simulink model "CMState"  (R2017b)
settings: Solver=VariableStepAuto  StartTime=0.0  StopTime=5  RelTol=1e-3
undefined symbols (not defined in the file or in its folder): Yo
settings Model: Creator=benma  LastModifiedBy=benma

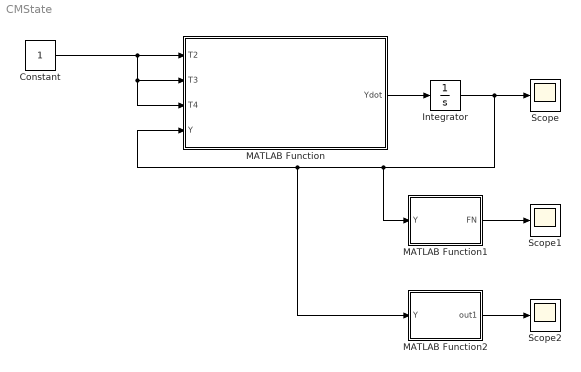
== system CMState ==
  Constant : Constant
  Integrator : Integrator  InitialCondition=Yo
  MATLAB Function : MATLAB Function  TreatAsAtomicUnit=on
  MATLAB Function1 : MATLAB Function  TreatAsAtomicUnit=on
  MATLAB Function2 : MATLAB Function  TreatAsAtomicUnit=on
  Scope : Scope
  Scope1 : Scope
  Scope2 : Scope
  wires:
  Integrator/1 -> Scope/1, MATLAB Function1/1(Y), MATLAB Function2/1(Y), MATLAB Function/4(Y)
  Constant/1 -> MATLAB Function/3(T4), MATLAB Function/2(T3), MATLAB Function/1(T2)
  MATLAB Function/1(Ydot) -> Integrator/1
  MATLAB Function1/1(FN) -> Scope1/1
  MATLAB Function2/1(out1) -> Scope2/1

== matlab function CMState/MATLAB Function ==
  data: T2 input; Ydot output; T3 input; T4 input; Y input
function Ydot = System1_ground(T2,T3,T4,Y)
%SYSTEM1_GROUND
%    OUT1 = SYSTEM1_GROUND(T2,T3,T4,Y)

%    This function was generated by the Symbolic Math Toolbox version 8.0.
%    22-Oct-2018 10:53:19

t2 = Y(2);
t3 = t2.*2.0;
t4 = Y(3);
t5 = t4.*2.0;
t6 = Y(4);
t7 = t6.*2.0;
t8 = Y(1);
t9 = Y(6);
t10 = t9.^2;
t11 = t2-t4;
t12 = sin(t11);
t13 = Y(7);
t14 = Y(8);
t15 = t2+t5;
t16 = sin(t15);
t17 = t13.^2;
t18 = t2-t7;
t19 = sin(t18);
t20 = t2+t7;
t21 = sin(t20);
t22 = cos(t5);
t23 = cos(t7);
t24 = -t2+t4+t7;
t25 = sin(t24);
t26 = t14.^2;
t27 = t2+t5+t7;
t28 = sin(t27);
t29 = cos(t15);
t30 = cos(t11);
t31 = cos(t18);
t32 = cos(t20);
t33 = cos(t27);
t34 = cos(t24);
t35 = t2+t4+t6;
t36 = sin(t35);
t37 = Y(9);
t38 = t3+t5;
t39 = t3-t7;
t40 = t3+t7;
t41 = t3+t5+t7;
t42 = sin(t2);
t43 = t5+t7;
t44 = cos(t43);
t45 = t2+t4;
t46 = sin(t45);
t47 = cos(t2);
t48 = -t2+t4+t6;
t49 = sin(t48);
t50 = t2-t4+t6;
t51 = sin(t50);
t52 = t2+t4-t6;
t53 = sin(t52);
t54 = t2+t4+t7;
t55 = sin(t54);
t56 = t37.^2;
t57 = cos(t45);
t58 = cos(t54);
t59 = cos(t41);
t60 = cos(t3);
t61 = cos(t38);
t62 = t61.*8.1e1;
t63 = cos(t39);
t64 = t63.*8.1e1;
t65 = cos(t40);
t66 = t65.*8.1e1;
t67 = t44.*4.5e1;
t191 = t59.*9.0;
t192 = t60.*6.57e2;
t193 = t22.*4.05e2;
t194 = t23.*3.33e2;
t68 = t62+t64+t66+t67-t191-t192-t193-t194+1.31e3;
t69 = 1.0./t68;
t70 = t5+t7-t8;
t71 = cos(t70);
t72 = cos(t8);
t73 = t3+t8;
t74 = cos(t73);
t75 = t74.*1.074195e5;
t76 = -t5+t8;
t77 = cos(t76);
t78 = t77.*3.97305e4;
t79 = t5+t8;
t80 = cos(t79);
t81 = t80.*3.97305e4;
t82 = -t7+t8;
t83 = cos(t82);
t84 = t83.*3.09015e4;
t85 = t7+t8;
t86 = cos(t85);
t87 = t86.*3.09015e4;
t88 = t3+t5+t8;
t89 = cos(t88);
t90 = t3-t7+t8;
t91 = cos(t90);
t92 = t3+t7+t8;
t93 = cos(t92);
t94 = t5+t7+t8;
t95 = cos(t94);
t96 = t3+t5+t7+t8;
t97 = cos(t96);
t98 = t97.*1.4715e3;
t99 = sin(t3);
t100 = sin(t5);
t101 = t10.*t12.*5.4e3;
t102 = t12.*t17.*5.4e3;
t103 = t12.*t26.*5.4e3;
t104 = t3+t4;
t105 = sin(t104);
t106 = t4-t6;
t107 = sin(t106);
t108 = t4+t7;
t109 = sin(t108);
t110 = T2.*t22.*8.1e3;
t111 = t10.*t25.*4.5e2;
t112 = t17.*t25.*4.5e2;
t113 = t3+t4-t6;
t114 = sin(t113);
t115 = t25.*t26.*4.5e2;
t116 = t3+t4+t7;
t117 = sin(t116);
t118 = t17.*t28.*1.5e2;
t119 = T3.*t30.*1.62e4;
t120 = cos(t104);
t121 = cos(t108);
t122 = T3.*t33.*9.0e2;
t123 = T4.*t34.*2.7e3;
t124 = cos(t116);
t125 = t10.*t36.*5.0e1;
t126 = t17.*t36.*5.0e1;
t127 = t26.*t36.*5.0e1;
t128 = t36.*t56.*5.0e1;
t129 = sin(t38);
t130 = sin(t39);
t131 = sin(t40);
t132 = sin(t43);
t133 = sin(t41);
t134 = t10.*t133.*1.5e2;
t135 = cos(t35);
t136 = t17.*t42.*1.87e4;
t137 = sin(t4);
t138 = t10.*t46.*3.15e3;
t139 = t17.*t46.*3.15e3;
t140 = t26.*t46.*3.15e3;
t141 = t4+t6;
t142 = sin(t141);
t143 = T3.*t47.*1.92e4;
t144 = cos(t4);
t145 = t10.*t51.*1.35e3;
t146 = t10.*t53.*9.0e2;
t147 = t17.*t51.*1.35e3;
t148 = t17.*t53.*9.0e2;
t149 = t26.*t51.*1.35e3;
t150 = t26.*t53.*9.0e2;
t151 = t3+t4+t6;
t152 = sin(t151);
t153 = t51.*t56.*1.35e3;
t154 = t53.*t56.*9.0e2;
t155 = T4.*t57.*1.35e4;
t156 = T3.*t58.*1.8e3;
t157 = cos(t48);
t158 = T4.*t157.*3.6e3;
t159 = cos(t50);
t160 = cos(t52);
t161 = T4.*t160.*5.4e3;
t162 = t9.*t13.*t46.*6.3e3;
t163 = t9.*t14.*t46.*6.3e3;
t164 = t13.*t14.*t46.*6.3e3;
t165 = t9.*t13.*t51.*2.7e3;
t166 = t9.*t13.*t53.*1.8e3;
t167 = t9.*t14.*t51.*2.7e3;
t168 = t9.*t14.*t53.*1.8e3;
t169 = t9.*t37.*t51.*2.7e3;
t170 = t13.*t14.*t51.*2.7e3;
t171 = t9.*t37.*t53.*1.8e3;
t172 = t13.*t14.*t53.*1.8e3;
t173 = t13.*t37.*t51.*2.7e3;
t174 = t13.*t37.*t53.*1.8e3;
t175 = t14.*t37.*t51.*2.7e3;
t176 = t14.*t37.*t53.*1.8e3;
t177 = t9.*t12.*t13.*1.08e4;
t178 = t9.*t12.*t14.*1.08e4;
t179 = t12.*t13.*t14.*1.08e4;
t180 = t9.*t13.*t25.*9.0e2;
t181 = t9.*t14.*t25.*9.0e2;
t182 = t9.*t13.*t28.*3.0e2;
t183 = t13.*t14.*t25.*9.0e2;
t184 = t9.*t13.*t36.*1.0e2;
t185 = t9.*t14.*t36.*1.0e2;
t186 = t9.*t36.*t37.*1.0e2;
t187 = t13.*t14.*t36.*1.0e2;
t188 = t13.*t36.*t37.*1.0e2;
t189 = t14.*t36.*t37.*1.0e2;
t190 = t9.*t13.*t42.*3.74e4;
t195 = t2+t8;
t196 = cos(t195);
t197 = t196.*1.702035e5;
t198 = t2+t5+t8;
t199 = cos(t198);
t200 = t2-t7+t8;
t201 = cos(t200);
t202 = t2+t7+t8;
t203 = cos(t202);
t204 = t2+t5+t7+t8;
t205 = cos(t204);
t206 = t205.*2.943e3;
t207 = -t2+t8;
t208 = cos(t207);
t209 = t2+t5-t8;
t210 = cos(t209);
t211 = t210.*3.97305e4;
t212 = t2+t7-t8;
t213 = cos(t212);
t214 = t213.*2.6487e4;
t215 = -t2+t7+t8;
t216 = cos(t215);
t217 = t216.*2.6487e4;
t218 = t2+t5+t7-t8;
t219 = cos(t218);
t220 = t10.*t99.*1.095e4;
t221 = t17.*t99.*1.095e4;
t222 = sin(t7);
t223 = t26.*t105.*5.4e3;
t224 = t3+t6;
t225 = sin(t224);
t226 = t5+t6;
t227 = sin(t226);
t228 = t26.*t109.*1.2e3;
t229 = t10.*t114.*1.35e3;
t230 = t17.*t114.*1.35e3;
t231 = t26.*t114.*1.35e3;
t232 = t3+t5+t6;
t233 = sin(t232);
t234 = t56.*t114.*1.35e3;
t235 = T2.*t29.*8.1e3;
t236 = T2.*t31.*2.7e3;
t237 = T2.*t32.*2.7e3;
t238 = T4.*t120.*1.62e4;
t239 = cos(t106);
t240 = T4.*t121.*7.2e3;
t241 = cos(t113);
t242 = T4.*t241.*8.1e3;
t243 = t3-t6;
t244 = sin(t243);
t245 = t10.*t132.*7.5e2;
t246 = t17.*t132.*7.5e2;
t247 = sin(t6);
t248 = T2.*t61.*8.1e3;
t249 = t10.*t152.*3.0e2;
t250 = t17.*t152.*3.0e2;
t251 = t26.*t152.*3.0e2;
t252 = t56.*t152.*3.0e2;
t253 = cos(t141);
t254 = T4.*t253.*1.41e4;
t255 = cos(t151);
t256 = t9.*t13.*t152.*6.0e2;
t257 = t9.*t14.*t152.*6.0e2;
t258 = t9.*t37.*t152.*6.0e2;
t259 = t13.*t14.*t152.*6.0e2;
t260 = t13.*t37.*t152.*6.0e2;
t261 = t14.*t37.*t152.*6.0e2;
t262 = t9.*t13.*t99.*2.19e4;
t263 = t9.*t14.*t105.*1.08e4;
t264 = t13.*t14.*t105.*1.08e4;
t265 = t9.*t14.*t109.*2.4e3;
t266 = t13.*t14.*t109.*2.4e3;
t267 = t9.*t13.*t114.*2.7e3;
t268 = t9.*t14.*t114.*2.7e3;
t269 = t9.*t37.*t114.*2.7e3;
t270 = t13.*t14.*t114.*2.7e3;
t271 = t13.*t37.*t114.*2.7e3;
t272 = t14.*t37.*t114.*2.7e3;
t273 = t9.*t13.*t132.*1.5e3;
t274 = t2+t4+t7+t8;
t275 = cos(t274);
t276 = t275.*1.4715e3;
t277 = t2+t4-t8;
t278 = cos(t277);
t279 = t278.*3.97305e4;
t280 = -t2+t4+t8;
t281 = cos(t280);
t282 = t2-t4+t8;
t283 = cos(t282);
t284 = t283.*5.2974e4;
t285 = t2+t4+t7-t8;
t286 = cos(t285);
t287 = -t2+t4+t7+t8;
t288 = cos(t287);
t289 = t288.*1.32435e4;
t290 = t2-t4-t7+t8;
t291 = cos(t290);
t292 = t2+t4+t8;
t293 = cos(t292);
t294 = t10.*t12.*1.35e4;
t295 = t10.*t25.*2.25e3;
t296 = t56.*t233.*4.5e2;
t297 = T2.*t120.*1.62e4;
t298 = T2.*t121.*7.2e3;
t299 = cos(t224);
t300 = cos(t226);
t301 = T2.*t34.*2.7e3;
t302 = cos(t232);
t303 = T3.*t124.*2.7e3;
t304 = t10.*t129.*1.35e3;
t305 = t17.*t129.*1.35e3;
t306 = t26.*t129.*1.35e3;
t307 = t56.*t244.*3.15e3;
t308 = t56.*t247.*1.19e4;
t309 = cos(t243);
t310 = T4.*t44.*4.5e3;
t311 = T3.*t59.*9.0e2;
t312 = T3.*t144.*2.97e4;
t313 = cos(t6);
t314 = t10.*t55.*6.0e2;
t315 = T2.*t57.*1.35e4;
t316 = t9.*t37.*t233.*9.0e2;
t317 = t13.*t37.*t233.*9.0e2;
t318 = t14.*t37.*t233.*9.0e2;
t319 = t9.*t13.*t129.*2.7e3;
t320 = t9.*t14.*t129.*2.7e3;
t321 = t13.*t14.*t129.*2.7e3;
t322 = t9.*t37.*t244.*6.3e3;
t323 = t13.*t37.*t244.*6.3e3;
t324 = t14.*t37.*t244.*6.3e3;
t325 = t9.*t37.*t247.*2.38e4;
t326 = t13.*t37.*t247.*2.38e4;
t327 = t14.*t37.*t247.*2.38e4;
Ydot = [t9;t13;t14;t37;Y(10);t69.*(T2.*-1.69e4-t71.*4.4145e3-t72.*2.418165e5+t75+t78+t81+t84+t87-t89.*1.32435e4-t91.*1.32435e4-t93.*1.32435e4-t95.*4.4145e3+t98+t101+t102+t103+t110+t111+t112+t115+t118+t119+t122+t123+t125+t126+t127+t128+t134+t136+t138+t139+t140+t143+t145+t146+t147+t148+t149+t150+t153+t154+t155+t156+t158+t161+t162+t163+t164+t165+t166+t167+t168+t169+t170+t171+t172+t173+t174+t175+t176+t177+t178+t179+t180+t181+t182+t183+t184+t185+t186+t187+t188+t189+t190+t220+t235+t236+t237+T2.*t23.*4.5e3-T3.*t29.*8.1e3-T3.*t31.*2.7e3-T4.*t30.*1.62e4-T2.*t33.*9.0e2-T3.*t32.*2.7e3-T3.*t34.*2.7e3-T2.*t44.*9.0e2-T2.*t47.*1.92e4-T3.*t57.*1.35e4-T4.*t58.*1.8e3-T4.*t135.*1.5e3-T4.*t159.*8.1e3-t10.*t16.*1.35e3-t10.*t19.*2.25e3-t10.*t21.*2.25e3-t16.*t17.*1.35e3-t17.*t19.*2.25e3+t10.*t28.*1.5e2-t17.*t21.*2.25e3+t10.*t42.*1.87e4-t10.*t49.*3.0e2-t10.*t55.*3.0e2-t17.*t49.*3.0e2-t17.*t55.*3.0e2-t26.*t49.*3.0e2-t26.*t55.*3.0e2-t49.*t56.*3.0e2-t10.*t129.*1.35e3-t10.*t130.*1.35e3-t10.*t131.*1.35e3-t9.*t13.*t16.*2.7e3-t9.*t13.*t19.*4.5e3-t9.*t13.*t21.*4.5e3-t9.*t13.*t49.*6.0e2-t9.*t14.*t49.*6.0e2-t13.*t14.*t49.*6.0e2-t9.*t13.*t55.*6.0e2-t9.*t14.*t55.*6.0e2-t13.*t14.*t55.*6.0e2-t9.*t37.*t49.*6.0e2-t13.*t37.*t49.*6.0e2-t14.*t37.*t49.*6.0e2).*(3.0./5.0e1);t69.*(T2.*-4.76e4+T3.*3.07e4-t71.*4.4145e3-t72.*2.418165e5+t75+t78+t81+t84+t87-t89.*1.32435e4-t91.*1.32435e4-t93.*1.32435e4-t95.*4.4145e3+t98+t101+t102+t103+t110+t111+t112+t115+t118+t119+t122+t123+t125+t126+t127+t128+t134+t136+t138+t139+t140+t143+t145+t146+t147+t148+t149+t150+t153+t154+t155+t156+t158+t161+t162+t163+t164+t165+t166+t167+t168+t169+t170+t171+t172+t173+t174+t175+t176+t177+t178+t179+t180+t181+t182+t183+t184+t185+t186+t187+t188+t189+t190+t197-t199.*2.6487e4-t201.*2.20725e4-t203.*2.20725e4+t206-t208.*2.015955e5+t211+t214+t217-t219.*4.4145e3+t221+t223+t228+t229+t230+t231+t234+t238+t240+t242+t245+t246+t248+t249+t250+t251+t252+t254+t256+t257+t258+t259+t260+t261+t262+t263+t264+t265+t266+t267+t268+t269+t270+t271+t272+t273+t303+t311+t312+T2.*t23.*1.44e4-T3.*t23.*9.9e3+T2.*t29.*1.62e4-T3.*t29.*8.1e3+T2.*t31.*5.4e3+T2.*t32.*5.4e3-T3.*t31.*2.7e3-T4.*t30.*1.62e4-T2.*t33.*1.8e3-T3.*t32.*2.7e3-T3.*t34.*2.7e3-T2.*t44.*9.0e2-T2.*t47.*3.84e4-T3.*t57.*1.35e4-T2.*t59.*9.0e2-T4.*t58.*1.8e3-T3.*t61.*8.1e3-T3.*t120.*1.62e4-T3.*t121.*7.2e3-T4.*t124.*2.7e3-T4.*t135.*1.5e3-T4.*t144.*2.97e4-T4.*t159.*8.1e3-T4.*t239.*2.16e4-T4.*t255.*3.6e3-t10.*t16.*8.1e3-t10.*t19.*7.2e3-t10.*t21.*7.2e3-t16.*t17.*1.35e3-t17.*t19.*2.25e3+t10.*t28.*9.0e2-t17.*t21.*2.25e3+t10.*t42.*5.66e4-t10.*t49.*3.0e2-t10.*t55.*3.0e2-t17.*t49.*3.0e2-t17.*t55.*3.0e2-t26.*t49.*3.0e2-t26.*t55.*3.0e2-t49.*t56.*3.0e2+t10.*t99.*2.19e4-t10.*t100.*6.75e3+t10.*t105.*5.4e3-t10.*t107.*3.6e3-t17.*t100.*6.75e3+t10.*t109.*1.2e3+t17.*t105.*5.4e3-t17.*t107.*3.6e3+t17.*t109.*1.2e3-t10.*t117.*4.5e2-t26.*t107.*3.6e3-t17.*t117.*4.5e2-t10.*t129.*1.35e3-t10.*t130.*2.7e3-t10.*t131.*2.7e3-t26.*t117.*4.5e2-t10.*t137.*1.665e4-t17.*t130.*1.35e3-t17.*t131.*1.35e3-t10.*t142.*1.55e3-t17.*t137.*1.665e4-t17.*t142.*1.55e3-t26.*t137.*1.665e4-t56.*t107.*3.6e3-t26.*t142.*1.55e3-t56.*t142.*1.55e3-t9.*t13.*t16.*2.7e3-t9.*t13.*t19.*4.5e3-t9.*t13.*t21.*4.5e3-t9.*t13.*t49.*6.0e2-t9.*t14.*t49.*6.0e2-t13.*t14.*t49.*6.0e2-t9.*t13.*t55.*6.0e2-t9.*t14.*t55.*6.0e2-t13.*t14.*t55.*6.0e2-t9.*t37.*t49.*6.0e2-t13.*t37.*t49.*6.0e2-t14.*t37.*t49.*6.0e2-t9.*t13.*t100.*1.35e4+t9.*t13.*t105.*1.08e4-t9.*t13.*t107.*7.2e3-t9.*t14.*t107.*7.2e3+t9.*t13.*t109.*2.4e3-t13.*t14.*t107.*7.2e3-t9.*t13.*t117.*9.0e2-t9.*t14.*t117.*9.0e2-t13.*t14.*t117.*9.0e2-t9.*t13.*t130.*2.7e3-t9.*t13.*t131.*2.7e3-t9.*t37.*t107.*7.2e3-t13.*t37.*t107.*7.2e3-t14.*t37.*t107.*7.2e3-t9.*t13.*t137.*3.33e4-t9.*t14.*t137.*3.33e4-t9.*t13.*t142.*3.1e3-t13.*t14.*t137.*3.33e4-t9.*t14.*t142.*3.1e3-t13.*t14.*t142.*3.1e3-t9.*t37.*t142.*3.1e3-t13.*t37.*t142.*3.1e3-t14.*t37.*t142.*3.1e3).*(-3.0./5.0e1);t69.*(T2.*-3.07e4+T3.*8.06e4-T4.*4.99e4+t197-t199.*2.6487e4-t201.*2.20725e4-t203.*2.20725e4+t206-t208.*2.015955e5+t211+t214+t217-t219.*4.4145e3+t220+t221+t223+t228+t229+t230+t231+t234+t235+t236+t237+t238+t240+t242+t245+t246+t248+t249+t250+t251+t252+t254+t256+t257+t258+t259+t260+t261+t262+t263+t264+t265+t266+t267+t268+t269+t270+t271+t272+t273+t276+t279-t281.*7.9461e4+t284-t286.*4.4145e3+t289-t291.*8.829e3-t293.*1.7658e4+t294+t295+t296+t297+t298+t301+t304+t305+t306+t307+t308+t310+t314+t315+t316+t317+t318+t319+t320+t321+t322+t323+t324+t325+t326+t327+T2.*t23.*9.9e3-T3.*t23.*9.9e3-T2.*t30.*1.62e4-T2.*t33.*9.0e2-T3.*t44.*4.5e3-T2.*t47.*1.92e4-T2.*t58.*1.8e3-T2.*t59.*9.0e2+T3.*t59.*1.8e3-T3.*t60.*3.15e4-T4.*t59.*9.0e2-T3.*t61.*8.1e3+T4.*t60.*3.15e4-T3.*t120.*3.24e4-T3.*t121.*1.44e4-T2.*t124.*2.7e3+T3.*t124.*5.4e3-T4.*t124.*2.7e3-T2.*t144.*2.97e4+T3.*t144.*5.94e4-T4.*t144.*2.97e4-T4.*t239.*2.16e4-T4.*t255.*3.6e3+T4.*t299.*1.35e4+T4.*t300.*1.35e4-T4.*t302.*2.7e3+T4.*t309.*1.35e4-T4.*t313.*4.92e4-t10.*t16.*6.75e3-t10.*t19.*4.95e3-t10.*t21.*4.95e3+t10.*t28.*7.5e2+t10.*t42.*3.79e4-t10.*t46.*5.85e3-t10.*t100.*1.35e4+t10.*t105.*8.1e3-t10.*t107.*3.6e3-t17.*t100.*1.35e4+t10.*t109.*4.5e3+t17.*t105.*8.1e3-t17.*t107.*3.6e3+t17.*t109.*4.5e3-t26.*t100.*6.75e3-t10.*t117.*9.0e2-t26.*t107.*3.6e3-t17.*t117.*9.0e2-t10.*t131.*2.7e3-t26.*t117.*4.5e2-t10.*t137.*3.87e4-t17.*t131.*2.7e3-t10.*t142.*1.55e3-t17.*t137.*3.87e4+t26.*t130.*1.35e3-t26.*t131.*1.35e3-t17.*t142.*1.55e3-t26.*t137.*1.665e4-t56.*t107.*3.6e3-t26.*t142.*1.55e3-t56.*t142.*1.55e3+t10.*t222.*5.55e3-t10.*t225.*3.15e3-t10.*t227.*2.25e3+t17.*t222.*5.55e3-t17.*t225.*3.15e3+t10.*t233.*4.5e2-t17.*t227.*2.25e3+t26.*t222.*5.55e3+t17.*t233.*4.5e2-t26.*t225.*3.15e3-t26.*t227.*2.25e3+t10.*t244.*3.15e3+t10.*t247.*1.19e4+t26.*t233.*4.5e2+t17.*t244.*3.15e3+t17.*t247.*1.19e4+t26.*t244.*3.15e3+t26.*t247.*1.19e4-t56.*t225.*3.15e3-t56.*t227.*2.25e3-t9.*t13.*t100.*2.7e4-t9.*t14.*t100.*1.35e4+t9.*t13.*t105.*1.62e4-t13.*t14.*t100.*1.35e4-t9.*t13.*t107.*7.2e3-t9.*t14.*t107.*7.2e3+t9.*t13.*t109.*9.0e3-t13.*t14.*t107.*7.2e3-t9.*t13.*t117.*1.8e3-t9.*t14.*t117.*9.0e2-t13.*t14.*t117.*9.0e2-t9.*t13.*t131.*5.4e3+t9.*t14.*t130.*2.7e3-t9.*t37.*t107.*7.2e3-t9.*t14.*t131.*2.7e3+t13.*t14.*t130.*2.7e3-t13.*t37.*t107.*7.2e3-t13.*t14.*t131.*2.7e3-t14.*t37.*t107.*7.2e3-t9.*t13.*t137.*7.74e4-t9.*t14.*t137.*3.33e4-t9.*t13.*t142.*3.1e3-t13.*t14.*t137.*3.33e4-t9.*t14.*t142.*3.1e3-t13.*t14.*t142.*3.1e3-t9.*t37.*t142.*3.1e3-t13.*t37.*t142.*3.1e3-t14.*t37.*t142.*3.1e3+t9.*t13.*t222.*1.11e4+t9.*t14.*t222.*1.11e4-t9.*t13.*t225.*6.3e3-t9.*t14.*t225.*6.3e3-t9.*t13.*t227.*4.5e3+t13.*t14.*t222.*1.11e4-t9.*t14.*t227.*4.5e3-t13.*t14.*t225.*6.3e3-t13.*t14.*t227.*4.5e3+t9.*t13.*t233.*9.0e2+t9.*t14.*t233.*9.0e2+t13.*t14.*t233.*9.0e2+t9.*t13.*t244.*6.3e3+t9.*t14.*t244.*6.3e3+t9.*t13.*t247.*2.38e4+t9.*t14.*t247.*2.38e4-t9.*t37.*t225.*6.3e3+t13.*t14.*t244.*6.3e3-t9.*t37.*t227.*4.5e3+t13.*t14.*t247.*2.38e4-t13.*t37.*t225.*6.3e3-t14.*t37.*t225.*6.3e3-t13.*t37.*t227.*4.5e3-t14.*t37.*t227.*4.5e3).*(3.0./5.0e1);t69.*(T3.*4.99e4-T4.*1.64e5+t125+t134+t229+t230-t245-t246+t267-t273+t276+t279-t281.*7.9461e4+t284-t286.*4.4145e3+t289-t291.*8.829e3-t293.*1.7658e4+t294+t295+t296+t297+t298+t301+t303+t304+t305+t306+t307+t308+t310+t311+t312+t314+t315+t316+t317+t318+t319+t320+t321+t322+t323+t324+t325+t326+t327-cos(t2-t4-t6+t8).*1.1772e4-cos(-t2+t4-t6+t8).*3.97305e4+cos(-t2-t4+t6+t8).*1.32435e4-cos(t2+t4+t6+t8).*9.81e2-cos(t2+t4+t6-t8).*1.4715e3-cos(t2+t4-t6+t8).*4.4145e3+cos(t2-t4+t6+t8).*2.6487e4+cos(-t2+t4+t6+t8).*1.7658e4+T4.*t22.*4.05e4-T2.*t30.*1.62e4-T3.*t44.*4.5e3-T2.*t58.*1.8e3-T3.*t60.*3.15e4-T4.*t59.*9.0e2+T4.*t60.*9.0e4-T4.*t61.*8.1e3-T3.*t120.*1.62e4-T3.*t121.*7.2e3-T2.*t124.*2.7e3-T2.*t135.*1.5e3-T2.*t144.*2.97e4+T2.*t157.*3.6e3-T2.*t159.*8.1e3+T2.*t160.*5.4e3-T2.*t239.*2.16e4+T3.*t239.*2.16e4+T2.*t241.*8.1e3-T3.*t241.*8.1e3+T2.*t253.*1.41e4-T3.*t253.*1.41e4-T2.*t255.*3.6e3+T3.*t255.*3.6e3-T3.*t299.*1.35e4-T3.*t300.*1.35e4+T4.*t299.*2.7e4+T4.*t300.*2.7e4+T3.*t302.*2.7e3-T4.*t302.*5.4e3-T3.*t309.*1.35e4+T4.*t309.*2.7e4+T3.*t313.*4.92e4-T4.*t313.*9.84e4-t10.*t46.*5.85e3+t10.*t49.*3.0e3+t10.*t51.*6.75e3-t10.*t53.*1.8e3-t10.*t100.*6.75e3+t10.*t105.*2.7e3-t10.*t107.*9.9e3-t17.*t100.*6.75e3+t10.*t109.*3.3e3+t17.*t105.*2.7e3-t17.*t107.*9.9e3+t17.*t109.*3.3e3-t26.*t100.*6.75e3-t10.*t117.*4.5e2-t17.*t117.*4.5e2+t10.*t130.*2.7e3-t10.*t131.*2.7e3-t10.*t137.*2.205e4+t17.*t130.*2.7e3-t17.*t131.*2.7e3+t17.*t133.*1.5e2+t10.*t142.*3.65e3-t17.*t137.*2.205e4+t26.*t130.*2.7e3-t26.*t131.*2.7e3-t26.*t132.*7.5e2+t17.*t142.*3.65e3+t26.*t133.*1.5e2-t10.*t152.*6.0e2-t17.*t152.*6.0e2+t56.*t130.*1.35e3-t56.*t131.*1.35e3-t56.*t132.*7.5e2+t56.*t133.*1.5e2+t10.*t222.*1.11e4-t10.*t225.*9.0e3-t10.*t227.*4.5e3+t17.*t222.*1.11e4-t17.*t225.*9.0e3+t10.*t233.*9.0e2-t17.*t227.*4.5e3+t26.*t222.*1.11e4+t17.*t233.*9.0e2-t26.*t225.*9.0e3-t26.*t227.*4.5e3+t10.*t244.*9.0e3+t10.*t247.*3.7e4+t26.*t233.*9.0e2+t17.*t244.*9.0e3+t17.*t247.*3.7e4+t26.*t244.*9.0e3+t26.*t247.*3.7e4+t56.*t222.*5.55e3-t56.*t225.*3.15e3-t56.*t227.*2.25e3-t9.*t13.*t100.*1.35e4-t9.*t14.*t100.*1.35e4+t9.*t13.*t105.*5.4e3-t13.*t14.*t100.*1.35e4-t9.*t13.*t107.*1.98e4+t9.*t13.*t109.*6.6e3-t9.*t13.*t117.*9.0e2+t9.*t13.*t130.*5.4e3-t9.*t13.*t131.*5.4e3+t9.*t14.*t130.*5.4e3-t9.*t14.*t131.*5.4e3+t9.*t13.*t133.*3.0e2-t9.*t14.*t132.*1.5e3+t9.*t14.*t133.*3.0e2+t13.*t14.*t130.*5.4e3-t13.*t14.*t131.*5.4e3-t9.*t13.*t137.*4.41e4-t13.*t14.*t132.*1.5e3+t13.*t14.*t133.*3.0e2+t9.*t13.*t142.*7.3e3-t9.*t13.*t152.*1.2e3+t9.*t37.*t130.*2.7e3-t9.*t37.*t131.*2.7e3-t9.*t37.*t132.*1.5e3+t9.*t37.*t133.*3.0e2+t13.*t37.*t130.*2.7e3-t13.*t37.*t131.*2.7e3+t14.*t37.*t130.*2.7e3-t13.*t37.*t132.*1.5e3-t14.*t37.*t131.*2.7e3+t13.*t37.*t133.*3.0e2-t14.*t37.*t132.*1.5e3+t14.*t37.*t133.*3.0e2+t9.*t13.*t222.*2.22e4+t9.*t14.*t222.*2.22e4-t9.*t13.*t225.*1.8e4-t9.*t14.*t225.*1.8e4-t9.*t13.*t227.*9.0e3+t13.*t14.*t222.*2.22e4-t9.*t14.*t227.*9.0e3-t13.*t14.*t225.*1.8e4-t13.*t14.*t227.*9.0e3+t9.*t13.*t233.*1.8e3+t9.*t14.*t233.*1.8e3+t13.*t14.*t233.*1.8e3+t9.*t13.*t244.*1.8e4+t9.*t14.*t244.*1.8e4+t9.*t37.*t222.*1.11e4+t9.*t13.*t247.*7.4e4+t9.*t14.*t247.*7.4e4-t9.*t37.*t225.*6.3e3+t13.*t14.*t244.*1.8e4+t13.*t37.*t222.*1.11e4-t9.*t37.*t227.*4.5e3+t14.*t37.*t222.*1.11e4+t13.*t14.*t247.*7.4e4-t13.*t37.*t225.*6.3e3-t14.*t37.*t225.*6.3e3-t13.*t37.*t227.*4.5e3-t14.*t37.*t227.*4.5e3).*(-3.0./5.0e1);0.0];

== matlab function CMState/MATLAB Function1 ==
  data: Y input; FN output
function FN = ground_force(Y)
%GROUND_FORCE
%    OUT1 = GROUND_FORCE(Y)

%    This function was generated by the Symbolic Math Toolbox version 8.0.
%    22-Oct-2018 11:02:05

t2 = Y(7);
t3 = Y(1);
t4 = Y(2);
t5 = Y(6);
t6 = Y(3);
t7 = Y(8);
t8 = Y(4);
t9 = t3+t4+t6+t8;
t10 = sin(t9);
t11 = Y(9);
t12 = t2+t5+t7+t11;
t13 = t10.*t12.*(1.0./2.0);
t14 = t3+t4;
t15 = sin(t14);
t16 = t2+t5;
t17 = t15.*t16.*(5.0./2.0);
t18 = t3+t4+t6;
t19 = sin(t18);
t20 = t2+t5+t7;
t21 = t19.*t20.*(3.0./2.0);
FN = -t7.*(t13+t21)-t5.*(t13+t17+t21+t5.*sin(t3).*(7.0./2.0))-t2.*(t13+t17+t21)-t10.*t11.*t12.*(1.0./2.0)+9.81e2./2.5e1;

== matlab function CMState/MATLAB Function2 ==
  data: Y input; out1 output
function out1 = center_of_mass_state(Y)
%CENTER_OF_MASS_STATE
%    OUT1 = CENTER_OF_MASS_STATE(Y)

%    This function was generated by the Symbolic Math Toolbox version 8.0.
%    22-Oct-2018 12:19:55

t2 = Y(1);
t3 = Y(2);
t4 = Y(3);
t5 = t2+t3;
t6 = Y(4);
t7 = t2+t3+t4+t6;
t8 = t2+t3+t4;
t9 = sin(t2);
t10 = sin(t7);
t11 = Y(6);
t12 = sin(t5);
t13 = Y(7);
t14 = sin(t8);
t15 = Y(8);
t16 = cos(t2);
t17 = cos(t7);
t18 = Y(9);
t19 = t11+t13+t15+t18;
t20 = cos(t5);
t21 = t11+t13;
t22 = cos(t8);
t23 = t11+t13+t15;
out1 = [t16.*(7.0./8.0)+t17.*(1.0./8.0)+t20.*(5.0./8.0)+t22.*(3.0./8.0);t9.*(7.0./8.0)+t10.*(1.0./8.0)+t12.*(5.0./8.0)+t14.*(3.0./8.0)+Y(5);t9.*t11.*(-7.0./8.0)-t10.*t19.*(1.0./8.0)-t12.*t21.*(5.0./8.0)-t14.*t23.*(3.0./8.0);t11.*t16.*(7.0./8.0)+t17.*t19.*(1.0./8.0)+t20.*t21.*(5.0./8.0)+t22.*t23.*(3.0./8.0)+Y(10)];
